simulink model "joystick"  (R2020a)
settings: Solver=VariableStepAuto  StartTime=0.0  StopTime=10.0  RelTol=1e-3
libraries: vrlib x1
settings Model: Creator=john  LastModifiedBy=john

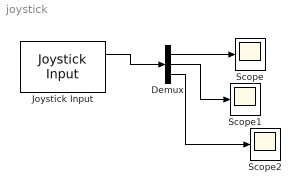
== system joystick ==
  Demux : Demux  Outputs=3
  Joystick Input : vrlib/Joystick Input  joyid=1  adjustports=on  forcefeed=off
  Scope : Scope
  Scope1 : Scope
  Scope2 : Scope
  wires:
  Joystick Input/1 -> Demux/1
  Demux/1 -> Scope/1
  Demux/2 -> Scope1/1
  Demux/3 -> Scope2/1
